simulink library "powerwindowlibdsp"  (Simulink 7.6)
settings: Solver=ode45  SolverMode=SingleTasking  StartTime=0.0  StopTime=10.0  RelTol=1e-3
libraries: powerlib x26, dspquant2 x6, simulink x4, xpclib x2
settings Model: Creator=The MathWorks Inc.  ExtModeAutoUpdateStatusClock=off

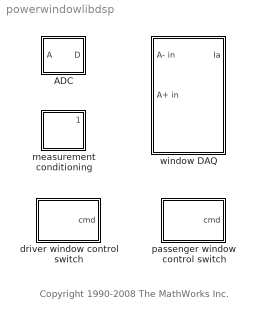
== system powerwindowlibdsp ==
  note: Copyright 1990-2008 The MathWorks Inc.
  ADC : Subsystem  mask(AD Converter){Ts=0.01, peak=3.5, Td=0.005, bits=8}
      mask prompts: Ts "sample time (-1 for inherited)"; Td "delay (-1 for inherited)"
      mask help: Analog (A) to digital (D) converter with sample rate, conversion delay, range, and number of bits used for conversion.
      mask Display:
      | plot([0.5 1.5 1.5 2.5 2.5 3.5 3.5 4.5], [0 0 1 1 2 2 3 3])
      | plot([0 3], [0 3])
  driver window control switch : Subsystem
  measurement conditioning : Subsystem
  passenger window control switch : Subsystem
  window DAQ : Subsystem

== system powerwindowlibdsp/ADC ==
  A : Inport
  Uniform Encoder : dspquant2/Uniform Encoder  peak=peak  bits=bits  otype=Signed integer
  Unit Delay : UnitDelay  SampleTime=Td
  Zero-Order Hold : ZeroOrderHold  SampleTime=Ts
  D : Outport
  wires:
  Uniform Encoder/1 -> D/1
  A/1 -> Unit Delay/1
  Unit Delay/1 -> Zero-Order Hold/1
  Zero-Order Hold/1 -> Uniform Encoder/1

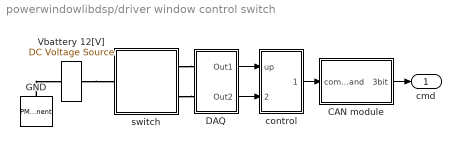
== system powerwindowlibdsp/driver window control switch ==
  CAN module : Subsystem
  DAQ : Subsystem
  GND : PMComponent  PhysicalDomain=powersysdomain  LeftPortType=p1  RightPortType=p1  LConnTagsString=a
      mask Type: Ground
      mask Description: Ground connection.
      mask Help: web(psbhelp);
      mask Display: plot(-10,-10,10,10,-[5 5],[-10 10],[0 0],[-5 5],-[-5 -5],[-2.5 2.5],-[15 5],[0 0])
  Vbattery 12[V] : powerlib/Electrical Sources/DC Voltage Source  SystemSampleTime=-1  Amplitude=12  Measurements=None
  control : Subsystem
  switch : Subsystem
  cmd : Outport
  wires:
  control/1(cmd) -> CAN module/1(command)
  CAN module/1(3bit) -> cmd/1
  DAQ/1(Out1) -> control/1(up)
  DAQ/2(Out2) -> control/2(down)
  connections:
  switch/RConn1 -- DAQ/LConn1
  switch/RConn2 -- DAQ/LConn2
  GND/LConn1 -- Vbattery 12[V]/LConn1
  Vbattery 12[V]/RConn1 -- switch/LConn1

== system powerwindowlibdsp/measurement conditioning ==
  R1 : powerlib/Elements/Series RLC Branch  DialogController=POWERSYS.PowerSysDialog  PhysicalDomain=powersysdomain  SubClassName=unknown  LeftPortType=p1  RightPortType=p1  LConnTagsString=__new0  RConnTagsString=__new0  BranchType=R  Resistance=0.18  Inductance=1.0  SetiL0=off  InitialCurrent=0  Capacitance=1.0  Setx0=off  InitialVoltage=0  Measurements=None
  measure1 : powerlib/Measurements/Voltage Measurement  DialogController=POWERSYS.PowerSysDialog  SystemSampleTime=-1  PhasorSimulation=off  OutputType=Magnitude  PSBequivalent=0
  Vin : PMIOPort  Tag=PMCPort  Port=1  Side=Left
  Vout : PMIOPort  Tag=PMCPort  Port=2  Side=Right
  Vmeas : Outport
  wires:
  measure1/1 -> Vmeas/1
  connections:
  Vout/RConn1 -- measure1/LConn2 -- R1/RConn1
  Vin/RConn1 -- R1/LConn1 -- measure1/LConn1

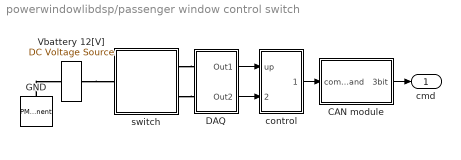
== system powerwindowlibdsp/passenger window control switch ==
  CAN module : Subsystem
  DAQ : Subsystem
  GND : PMComponent  PhysicalDomain=powersysdomain  LeftPortType=p1  RightPortType=p1  LConnTagsString=a
      mask Type: Ground
      mask Description: Ground connection.
      mask Help: web(psbhelp);
      mask Display: plot(-10,-10,10,10,-[5 5],[-10 10],[0 0],[-5 5],-[-5 -5],[-2.5 2.5],-[15 5],[0 0])
  Vbattery 12[V] : powerlib/Electrical Sources/DC Voltage Source  SystemSampleTime=-1  Amplitude=12  Measurements=None
  control : Subsystem
  switch : Subsystem
  cmd : Outport
  wires:
  DAQ/2(Out2) -> control/2(down)
  DAQ/1(Out1) -> control/1(up)
  CAN module/1(3bit) -> cmd/1
  control/1(cmd) -> CAN module/1(command)
  connections:
  Vbattery 12[V]/RConn1 -- switch/LConn1
  GND/LConn1 -- Vbattery 12[V]/LConn1
  switch/RConn2 -- DAQ/LConn2
  switch/RConn1 -- DAQ/LConn1

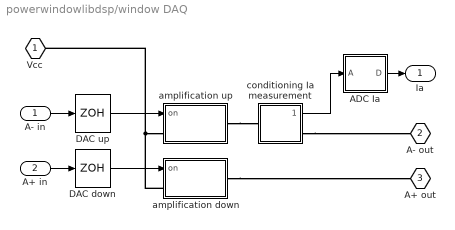
== system powerwindowlibdsp/window DAQ ==
  A- in : Inport
  A+ in : Inport  Port=2
  ADC Ia : Subsystem  mask(AD Converter){Ts=0.01, peak=3.5, Td=0.005, bits=8}
      mask prompts: Ts "sample time (-1 for inherited)"; Td "delay (-1 for inherited)"
      mask help: Analog (A) to digital (D) converter with sample rate, conversion delay, range, and number of bits used for conversion.
      mask Display:
      | plot([0.5 1.5 1.5 2.5 2.5 3.5 3.5 4.5], [0 0 1 1 2 2 3 3])
      | plot([0 3], [0 3])
  DAC down : ZeroOrderHold  SampleTime=0.01
  DAC up : ZeroOrderHold  SampleTime=0.01
  amplification down : Subsystem
  amplification up : Subsystem
  conditioning Ia measurement : Subsystem
  Vcc : PMIOPort  Port=1  Side=Left
  A- out : PMIOPort  Port=2  Side=Right
  A+ out : PMIOPort  Port=3  Side=Right
  Ia : Outport
  wires:
  DAC up/1 -> amplification up/1(on)
  DAC down/1 -> amplification down/1(on)
  conditioning Ia measurement/1(Vmeas) -> ADC Ia/1(A)
  ADC Ia/1(D) -> Ia/1
  A- in/1 -> DAC up/1
  A+ in/1 -> DAC down/1
  connections:
  amplification down/LConn1 -- Vcc/RConn1 -- amplification up/LConn1
  amplification up/RConn1 -- conditioning Ia measurement/LConn1
  conditioning Ia measurement/RConn1 -- A- out/RConn1
  amplification down/RConn1 -- A+ out/RConn1

== system powerwindowlibdsp/driver window control switch/CAN module ==
  command : Inport
  "CAN bit-packing " : xpclib/CAN/Utilities/CAN bit-packing   bitpatterns={ [0:0] [1:1] [2:2]}
  Demux : Demux  Outputs=3
  3bit : Outport
  wires:
  "CAN bit-packing "/1 -> 3bit/1
  command/1 -> Demux/1
  Demux/1 -> "CAN bit-packing "/1
  Demux/2 -> "CAN bit-packing "/2
  Demux/3 -> "CAN bit-packing "/3

== system powerwindowlibdsp/driver window control switch/DAQ ==
  DAQ driver down : Subsystem
  DAQ driver up : Subsystem
  In1 : PMIOPort  Port=1  Side=Left
  In2 : PMIOPort  Port=2  Side=Left
  Out1 : Outport
  Out2 : Outport  Port=2
  wires:
  DAQ driver up/1(active) -> Out1/1
  DAQ driver down/1(active) -> Out2/1
  connections:
  In1/RConn1 -- DAQ driver up/LConn1
  In2/RConn1 -- DAQ driver down/LConn1

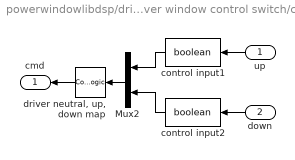
== system powerwindowlibdsp/driver window control switch/control ==
  up : Inport
  down : Inport  Port=2
  Mux2 : Mux  Inputs=2
  control input1 : DataTypeConversion  OutDataTypeStr=boolean  SaturateOnIntegerOverflow=on  RndMeth=Zero
  control input2 : DataTypeConversion  OutDataTypeStr=boolean  SaturateOnIntegerOverflow=on  RndMeth=Zero
  "driver neutral, up, down map" : CombinatorialLogic  TruthTable=[1 0 0;0 0 1;0 1 0;1 0 0]
  cmd : Outport
  wires:
  Mux2/1 -> "driver neutral, up, down map"/1
  control input1/1 -> Mux2/1
  control input2/1 -> Mux2/2
  up/1 -> control input1/1
  "driver neutral, up, down map"/1 -> cmd/1
  down/1 -> control input2/1

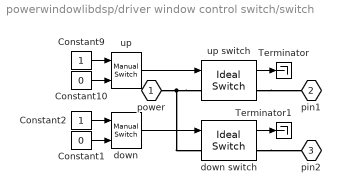
== system powerwindowlibdsp/driver window control switch/switch ==
  Constant1 : Constant  Value=0
  Constant10 : Constant  Value=0
  Constant2 : Constant
  Constant9 : Constant
  Terminator : Terminator
  Terminator1 : Terminator
  down : simulink/Signal Routing/Manual Switch  SystemSampleTime=-1  sw=0  action=0
  down switch : powerlib/Power Electronics/Ideal Switch  SystemSampleTime=-1  Ron=0.01  Lon=0  IC=0  Rs=1000000  Cs=inf  Measurements=on
  up : simulink/Signal Routing/Manual Switch  SystemSampleTime=-1  sw=0  action=0
  up switch : powerlib/Power Electronics/Ideal Switch  SystemSampleTime=-1  Ron=0.01  Lon=0  IC=0  Rs=1000000  Cs=inf  Measurements=on
  power : PMIOPort  Port=1  Side=Left
  pin1 : PMIOPort  Port=2  Side=Right
  pin2 : PMIOPort  Port=3  Side=Right
  wires:
  down/1 -> down switch/1
  down switch/1 -> Terminator1/1
  up/1 -> up switch/1
  up switch/1 -> Terminator/1
  Constant1/1 -> down/2
  Constant2/1 -> down/1
  Constant10/1 -> up/2
  Constant9/1 -> up/1
  connections:
  up switch/LConn1 -- power/RConn1 -- down switch/LConn1
  down switch/RConn1 -- pin2/RConn1
  up switch/RConn1 -- pin1/RConn1

== system powerwindowlibdsp/passenger window control switch/CAN module ==
  command : Inport
  "CAN bit-packing " : xpclib/CAN/Utilities/CAN bit-packing   bitpatterns={ [0:0] [1:1] [2:2]}
  Demux : Demux  Outputs=3
  3bit : Outport
  wires:
  Demux/3 -> "CAN bit-packing "/3
  Demux/2 -> "CAN bit-packing "/2
  Demux/1 -> "CAN bit-packing "/1
  command/1 -> Demux/1
  "CAN bit-packing "/1 -> 3bit/1

== system powerwindowlibdsp/passenger window control switch/DAQ ==
  DAQ driver down : Subsystem
  DAQ driver up : Subsystem
  In1 : PMIOPort  Port=1  Side=Left
  In2 : PMIOPort  Port=2  Side=Left
  Out1 : Outport
  Out2 : Outport  Port=2
  wires:
  DAQ driver down/1(active) -> Out2/1
  DAQ driver up/1(active) -> Out1/1
  connections:
  In2/RConn1 -- DAQ driver down/LConn1
  In1/RConn1 -- DAQ driver up/LConn1

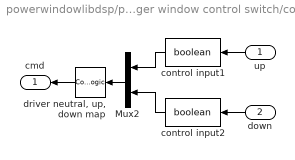
== system powerwindowlibdsp/passenger window control switch/control ==
  up : Inport
  down : Inport  Port=2
  Mux2 : Mux  Inputs=2
  control input1 : DataTypeConversion  OutDataTypeStr=boolean  SaturateOnIntegerOverflow=on  RndMeth=Zero
  control input2 : DataTypeConversion  OutDataTypeStr=boolean  SaturateOnIntegerOverflow=on  RndMeth=Zero
  "driver neutral, up, down map" : CombinatorialLogic  TruthTable=[1 0 0;0 0 1;0 1 0;1 0 0]
  cmd : Outport
  wires:
  down/1 -> control input2/1
  "driver neutral, up, down map"/1 -> cmd/1
  up/1 -> control input1/1
  control input2/1 -> Mux2/2
  control input1/1 -> Mux2/1
  Mux2/1 -> "driver neutral, up, down map"/1

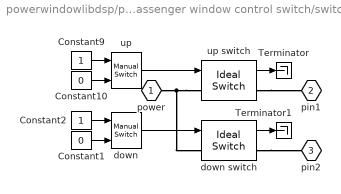
== system powerwindowlibdsp/passenger window control switch/switch ==
  Constant1 : Constant  Value=0
  Constant10 : Constant  Value=0
  Constant2 : Constant
  Constant9 : Constant
  Terminator : Terminator
  Terminator1 : Terminator
  down : simulink/Signal Routing/Manual Switch  SystemSampleTime=-1  sw=0  action=0
  down switch : powerlib/Power Electronics/Ideal Switch  SystemSampleTime=-1  Ron=0.01  Lon=0  IC=0  Rs=1000000  Cs=inf  Measurements=on
  up : simulink/Signal Routing/Manual Switch  SystemSampleTime=-1  sw=0  action=0
  up switch : powerlib/Power Electronics/Ideal Switch  SystemSampleTime=-1  Ron=0.01  Lon=0  IC=0  Rs=1000000  Cs=inf  Measurements=on
  power : PMIOPort  Port=1  Side=Left
  pin1 : PMIOPort  Port=2  Side=Right
  pin2 : PMIOPort  Port=3  Side=Right
  wires:
  Constant9/1 -> up/1
  Constant10/1 -> up/2
  Constant2/1 -> down/1
  Constant1/1 -> down/2
  up switch/1 -> Terminator/1
  up/1 -> up switch/1
  down switch/1 -> Terminator1/1
  down/1 -> down switch/1
  connections:
  up switch/RConn1 -- pin1/RConn1
  down switch/RConn1 -- pin2/RConn1
  up switch/LConn1 -- down switch/LConn1 -- power/RConn1

== system powerwindowlibdsp/window DAQ/ADC Ia ==
  A : Inport
  Uniform Encoder : dspquant2/Uniform Encoder  peak=peak  bits=bits  otype=Signed integer
  Unit Delay : UnitDelay  SampleTime=Td
  Zero-Order Hold : ZeroOrderHold  SampleTime=Ts
  D : Outport
  wires:
  Uniform Encoder/1 -> D/1
  A/1 -> Unit Delay/1
  Unit Delay/1 -> Zero-Order Hold/1
  Zero-Order Hold/1 -> Uniform Encoder/1

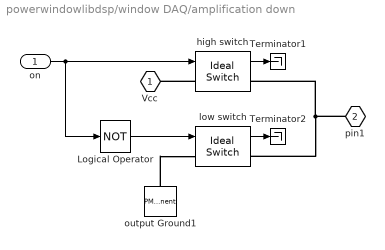
== system powerwindowlibdsp/window DAQ/amplification down ==
  on : Inport
  Logical Operator : Logic  Operator=NOT
  Terminator1 : Terminator
  Terminator2 : Terminator
  high switch : powerlib/Power Electronics/Ideal Switch  DialogController=POWERSYS.PowerSysDialog  SystemSampleTime=-1  Ron=0.01  Lon=0  IC=0  Rs=1000000  Cs=inf  Measurements=on
  low switch : powerlib/Power Electronics/Ideal Switch  DialogController=POWERSYS.PowerSysDialog  SystemSampleTime=-1  Ron=0.01  Lon=0  IC=0  Rs=1000000  Cs=inf  Measurements=on
  output Ground1 : PMComponent  PhysicalDomain=powersysdomain  LeftPortType=p1  RightPortType=p1  LConnTagsString=a
      mask Type: Ground
      mask Description: Ground connection.
      mask Help: web(psbhelp);
      mask Display: plot(-10,-10,10,10,-[5 5],[-10 10],[0 0],[-5 5],-[-5 -5],[-2.5 2.5],-[15 5],[0 0])
  Vcc : PMIOPort  Port=1  Side=Left
  pin1 : PMIOPort  Port=2  Side=Right
  wires:
  low switch/1 -> Terminator2/1
  on/1 -> Logical Operator/1, high switch/1
  high switch/1 -> Terminator1/1
  Logical Operator/1 -> low switch/1
  connections:
  high switch/LConn1 -- Vcc/RConn1
  output Ground1/LConn1 -- low switch/LConn1
  low switch/RConn1 -- high switch/RConn1 -- pin1/RConn1

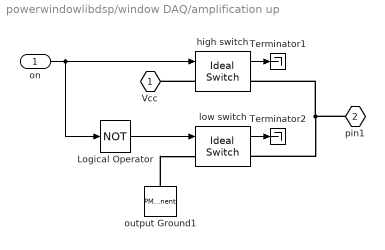
== system powerwindowlibdsp/window DAQ/amplification up ==
  on : Inport
  Logical Operator : Logic  Operator=NOT
  Terminator1 : Terminator
  Terminator2 : Terminator
  high switch : powerlib/Power Electronics/Ideal Switch  DialogController=POWERSYS.PowerSysDialog  SystemSampleTime=-1  Ron=0.01  Lon=0  IC=0  Rs=1000000  Cs=inf  Measurements=on
  low switch : powerlib/Power Electronics/Ideal Switch  SystemSampleTime=-1  Ron=0.01  Lon=0  IC=0  Rs=1000000  Cs=inf  Measurements=on
  output Ground1 : PMComponent  PhysicalDomain=powersysdomain  LeftPortType=p1  RightPortType=p1  LConnTagsString=a
      mask Type: Ground
      mask Description: Ground connection.
      mask Help: web(psbhelp);
      mask Display: plot(-10,-10,10,10,-[5 5],[-10 10],[0 0],[-5 5],-[-5 -5],[-2.5 2.5],-[15 5],[0 0])
  Vcc : PMIOPort  Port=1  Side=Left
  pin1 : PMIOPort  Port=2  Side=Right
  wires:
  low switch/1 -> Terminator2/1
  on/1 -> high switch/1, Logical Operator/1
  high switch/1 -> Terminator1/1
  Logical Operator/1 -> low switch/1
  connections:
  high switch/RConn1 -- low switch/RConn1 -- pin1/RConn1
  high switch/LConn1 -- Vcc/RConn1
  output Ground1/LConn1 -- low switch/LConn1

== system powerwindowlibdsp/window DAQ/conditioning Ia measurement ==
  R1 : powerlib/Elements/Series RLC Branch  DialogController=POWERSYS.PowerSysDialog  PhysicalDomain=powersysdomain  SubClassName=unknown  LeftPortType=p1  RightPortType=p1  LConnTagsString=__new0  RConnTagsString=__new0  BranchType=R  Resistance=0.18  Inductance=1.0  SetiL0=off  InitialCurrent=0  Capacitance=1.0  Setx0=off  InitialVoltage=0  Measurements=None
  measure1 : powerlib/Measurements/Voltage Measurement  DialogController=POWERSYS.PowerSysDialog  SystemSampleTime=-1  PhasorSimulation=off  OutputType=Magnitude  PSBequivalent=0
  Vin : PMIOPort  Port=1  Side=Left
  Vout : PMIOPort  Port=2  Side=Right
  Vmeas : Outport
  wires:
  measure1/1 -> Vmeas/1
  connections:
  measure1/LConn2 -- Vout/RConn1 -- R1/RConn1
  R1/LConn1 -- measure1/LConn1 -- Vin/RConn1

== system powerwindowlibdsp/driver window control switch/DAQ/DAQ driver down ==
  ADC driver up : Subsystem  mask(AD Converter){Ts=0.01, Td=0.005, peak=4.9, bits=2}
      mask prompts: Ts "sample time (-1 for inherited)"; Td "delay (-1 for inherited)"
      mask help: Analog (A) to digital (D) converter with sample rate, conversion delay, range, and number of bits used for conversion.
      mask init:
      | gain = peak / (2^(bits-1));
      mask Display:
      | plot([0.5 1.5 1.5 2.5 2.5 3.5 3.5 4.5], [0 0 1 1 2 2 3 3])
      | plot([0 3], [0 3])
  conditioning driver up : Subsystem
  Vin : PMIOPort  Port=1  Side=Left
  active : Outport
  wires:
  ADC driver up/1(D) -> active/1
  conditioning driver up/1(active) -> ADC driver up/1(A)
  connections:
  Vin/RConn1 -- conditioning driver up/LConn1

== system powerwindowlibdsp/driver window control switch/DAQ/DAQ driver up ==
  ADC driver up : Subsystem  mask(AD Converter){Ts=0.01, Td=0.005, peak=4.9, bits=2}
      mask prompts: Ts "sample time (-1 for inherited)"; Td "delay (-1 for inherited)"
      mask help: Analog (A) to digital (D) converter with sample rate, conversion delay, range, and number of bits used for conversion.
      mask init:
      | gain = peak / (2^(bits-1));
      mask Display:
      | plot([0.5 1.5 1.5 2.5 2.5 3.5 3.5 4.5], [0 0 1 1 2 2 3 3])
      | plot([0 3], [0 3])
  conditioning driver up : Subsystem
  Vin : PMIOPort  Port=1  Side=Left
  active : Outport
  wires:
  conditioning driver up/1(active) -> ADC driver up/1(A)
  ADC driver up/1(D) -> active/1
  connections:
  Vin/RConn1 -- conditioning driver up/LConn1

== system powerwindowlibdsp/passenger window control switch/DAQ/DAQ driver down ==
  ADC driver up : Subsystem  mask(AD Converter){Ts=0.01, Td=0.005, peak=4.9, bits=2}
      mask prompts: Ts "sample time (-1 for inherited)"; Td "delay (-1 for inherited)"
      mask help: Analog (A) to digital (D) converter with sample rate, conversion delay, range, and number of bits used for conversion.
      mask init:
      | gain = peak / (2^(bits-1));
      mask Display:
      | plot([0.5 1.5 1.5 2.5 2.5 3.5 3.5 4.5], [0 0 1 1 2 2 3 3])
      | plot([0 3], [0 3])
  conditioning driver up : Subsystem
  Vin : PMIOPort  Port=1  Side=Left
  active : Outport
  wires:
  conditioning driver up/1(active) -> ADC driver up/1(A)
  ADC driver up/1(D) -> active/1
  connections:
  Vin/RConn1 -- conditioning driver up/LConn1

== system powerwindowlibdsp/passenger window control switch/DAQ/DAQ driver up ==
  ADC driver up : Subsystem  mask(AD Converter){Ts=0.01, Td=0.005, peak=4.9, bits=2}
      mask prompts: Ts "sample time (-1 for inherited)"; Td "delay (-1 for inherited)"
      mask help: Analog (A) to digital (D) converter with sample rate, conversion delay, range, and number of bits used for conversion.
      mask init:
      | gain = peak / (2^(bits-1));
      mask Display:
      | plot([0.5 1.5 1.5 2.5 2.5 3.5 3.5 4.5], [0 0 1 1 2 2 3 3])
      | plot([0 3], [0 3])
  conditioning driver up : Subsystem
  Vin : PMIOPort  Port=1  Side=Left
  active : Outport
  wires:
  ADC driver up/1(D) -> active/1
  conditioning driver up/1(active) -> ADC driver up/1(A)
  connections:
  Vin/RConn1 -- conditioning driver up/LConn1

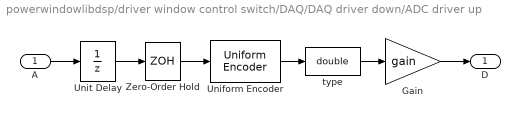
== system powerwindowlibdsp/driver window control switch/DAQ/DAQ driver down/ADC driver up ==
  A : Inport
  Gain : Gain  Gain=gain  SaturateOnIntegerOverflow=on  OutDataTypeStr=Inherit: Same as input  ParamDataTypeStr=Inherit: Same as input
  Uniform Encoder : dspquant2/Uniform Encoder  peak=peak  bits=bits  otype=Signed integer
  Unit Delay : UnitDelay  SampleTime=Td
  Zero-Order Hold : ZeroOrderHold  SampleTime=Ts
  type : DataTypeConversion  OutDataTypeStr=double  SaturateOnIntegerOverflow=on  RndMeth=Zero
  D : Outport
  wires:
  Zero-Order Hold/1 -> Uniform Encoder/1
  Unit Delay/1 -> Zero-Order Hold/1
  A/1 -> Unit Delay/1
  Uniform Encoder/1 -> type/1
  type/1 -> Gain/1
  Gain/1 -> D/1

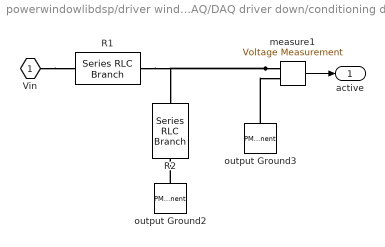
== system powerwindowlibdsp/driver window control switch/DAQ/DAQ driver down/conditioning driver up ==
  R1 : powerlib/Elements/Series RLC Branch  PhysicalDomain=powersysdomain  SubClassName=unknown  LeftPortType=p1  RightPortType=p1  LConnTagsString=__new0  RConnTagsString=__new0  BranchType=R  Resistance=6800  Inductance=1.0  SetiL0=off  InitialCurrent=0  Capacitance=1.0  Setx0=off  InitialVoltage=0  Measurements=None
  R2 : powerlib/Elements/Series RLC Branch  PhysicalDomain=powersysdomain  SubClassName=unknown  LeftPortType=p1  RightPortType=p1  LConnTagsString=__new0  RConnTagsString=__new0  BranchType=R  Resistance=4700  Inductance=1.0  SetiL0=off  InitialCurrent=0  Capacitance=1.0  Setx0=off  InitialVoltage=0  Measurements=None
  measure1 : powerlib/Measurements/Voltage Measurement  SystemSampleTime=-1  PhasorSimulation=off  OutputType=Magnitude  PSBequivalent=0
  output Ground2 : PMComponent  PhysicalDomain=powersysdomain  LeftPortType=p1  RightPortType=p1  LConnTagsString=a
      mask Type: Ground
      mask Description: Ground connection.
      mask Help: web(psbhelp);
      mask Display: plot(-10,-10,10,10,-[5 5],[-10 10],[0 0],[-5 5],-[-5 -5],[-2.5 2.5],-[15 5],[0 0])
  output Ground3 : PMComponent  PhysicalDomain=powersysdomain  LeftPortType=p1  RightPortType=p1  LConnTagsString=a
      mask Type: Ground
      mask Description: Ground connection.
      mask Help: web(psbhelp);
      mask Display: plot(-10,-10,10,10,-[5 5],[-10 10],[0 0],[-5 5],-[-5 -5],[-2.5 2.5],-[15 5],[0 0])
  Vin : PMIOPort  Port=1  Side=Left
  active : Outport
  wires:
  measure1/1 -> active/1
  connections:
  output Ground3/LConn1 -- measure1/LConn2
  output Ground2/LConn1 -- R2/LConn1
  Vin/RConn1 -- R1/LConn1
  measure1/LConn1 -- R2/RConn1 -- R1/RConn1

== system powerwindowlibdsp/driver window control switch/DAQ/DAQ driver up/ADC driver up ==
  A : Inport
  Gain : Gain  Gain=gain  SaturateOnIntegerOverflow=on  OutDataTypeStr=Inherit: Same as input  ParamDataTypeStr=Inherit: Same as input
  Uniform Encoder : dspquant2/Uniform Encoder  peak=peak  bits=bits  otype=Signed integer
  Unit Delay : UnitDelay  SampleTime=Td
  Zero-Order Hold : ZeroOrderHold  SampleTime=Ts
  type : DataTypeConversion  OutDataTypeStr=double  SaturateOnIntegerOverflow=on  RndMeth=Zero
  D : Outport
  wires:
  Gain/1 -> D/1
  type/1 -> Gain/1
  Uniform Encoder/1 -> type/1
  A/1 -> Unit Delay/1
  Unit Delay/1 -> Zero-Order Hold/1
  Zero-Order Hold/1 -> Uniform Encoder/1

== system powerwindowlibdsp/driver window control switch/DAQ/DAQ driver up/conditioning driver up ==
  R1 : powerlib/Elements/Series RLC Branch  PhysicalDomain=powersysdomain  SubClassName=unknown  LeftPortType=p1  RightPortType=p1  LConnTagsString=__new0  RConnTagsString=__new0  BranchType=R  Resistance=6800  Inductance=1.0  SetiL0=off  InitialCurrent=0  Capacitance=1.0  Setx0=off  InitialVoltage=0  Measurements=None
  R2 : powerlib/Elements/Series RLC Branch  PhysicalDomain=powersysdomain  SubClassName=unknown  LeftPortType=p1  RightPortType=p1  LConnTagsString=__new0  RConnTagsString=__new0  BranchType=R  Resistance=4700  Inductance=1.0  SetiL0=off  InitialCurrent=0  Capacitance=1.0  Setx0=off  InitialVoltage=0  Measurements=None
  measure1 : powerlib/Measurements/Voltage Measurement  SystemSampleTime=-1  PhasorSimulation=off  OutputType=Magnitude  PSBequivalent=0
  output Ground2 : PMComponent  PhysicalDomain=powersysdomain  LeftPortType=p1  RightPortType=p1  LConnTagsString=a
      mask Type: Ground
      mask Description: Ground connection.
      mask Help: web(psbhelp);
      mask Display: plot(-10,-10,10,10,-[5 5],[-10 10],[0 0],[-5 5],-[-5 -5],[-2.5 2.5],-[15 5],[0 0])
  output Ground3 : PMComponent  PhysicalDomain=powersysdomain  LeftPortType=p1  RightPortType=p1  LConnTagsString=a
      mask Type: Ground
      mask Description: Ground connection.
      mask Help: web(psbhelp);
      mask Display: plot(-10,-10,10,10,-[5 5],[-10 10],[0 0],[-5 5],-[-5 -5],[-2.5 2.5],-[15 5],[0 0])
  Vin : PMIOPort  Port=1  Side=Left
  active : Outport
  wires:
  measure1/1 -> active/1
  connections:
  measure1/LConn1 -- R1/RConn1 -- R2/RConn1
  Vin/RConn1 -- R1/LConn1
  output Ground2/LConn1 -- R2/LConn1
  output Ground3/LConn1 -- measure1/LConn2

== system powerwindowlibdsp/passenger window control switch/DAQ/DAQ driver down/ADC driver up ==
  A : Inport
  Gain : Gain  Gain=gain  SaturateOnIntegerOverflow=on  OutDataTypeStr=Inherit: Same as input  ParamDataTypeStr=Inherit: Same as input
  Uniform Encoder : dspquant2/Uniform Encoder  peak=peak  bits=bits  otype=Signed integer
  Unit Delay : UnitDelay  SampleTime=Td
  Zero-Order Hold : ZeroOrderHold  SampleTime=Ts
  type : DataTypeConversion  OutDataTypeStr=double  SaturateOnIntegerOverflow=on  RndMeth=Zero
  D : Outport
  wires:
  Gain/1 -> D/1
  type/1 -> Gain/1
  Uniform Encoder/1 -> type/1
  A/1 -> Unit Delay/1
  Unit Delay/1 -> Zero-Order Hold/1
  Zero-Order Hold/1 -> Uniform Encoder/1

== system powerwindowlibdsp/passenger window control switch/DAQ/DAQ driver down/conditioning driver up ==
  R1 : powerlib/Elements/Series RLC Branch  PhysicalDomain=powersysdomain  SubClassName=unknown  LeftPortType=p1  RightPortType=p1  LConnTagsString=__new0  RConnTagsString=__new0  BranchType=R  Resistance=6800  Inductance=1.0  SetiL0=off  InitialCurrent=0  Capacitance=1.0  Setx0=off  InitialVoltage=0  Measurements=None
  R2 : powerlib/Elements/Series RLC Branch  PhysicalDomain=powersysdomain  SubClassName=unknown  LeftPortType=p1  RightPortType=p1  LConnTagsString=__new0  RConnTagsString=__new0  BranchType=R  Resistance=4700  Inductance=1.0  SetiL0=off  InitialCurrent=0  Capacitance=1.0  Setx0=off  InitialVoltage=0  Measurements=None
  measure1 : powerlib/Measurements/Voltage Measurement  SystemSampleTime=-1  PhasorSimulation=off  OutputType=Magnitude  PSBequivalent=0
  output Ground2 : PMComponent  PhysicalDomain=powersysdomain  LeftPortType=p1  RightPortType=p1  LConnTagsString=a
      mask Type: Ground
      mask Description: Ground connection.
      mask Help: web(psbhelp);
      mask Display: plot(-10,-10,10,10,-[5 5],[-10 10],[0 0],[-5 5],-[-5 -5],[-2.5 2.5],-[15 5],[0 0])
  output Ground3 : PMComponent  PhysicalDomain=powersysdomain  LeftPortType=p1  RightPortType=p1  LConnTagsString=a
      mask Type: Ground
      mask Description: Ground connection.
      mask Help: web(psbhelp);
      mask Display: plot(-10,-10,10,10,-[5 5],[-10 10],[0 0],[-5 5],-[-5 -5],[-2.5 2.5],-[15 5],[0 0])
  Vin : PMIOPort  Port=1  Side=Left
  active : Outport
  wires:
  measure1/1 -> active/1
  connections:
  R1/RConn1 -- R2/RConn1 -- measure1/LConn1
  Vin/RConn1 -- R1/LConn1
  output Ground2/LConn1 -- R2/LConn1
  output Ground3/LConn1 -- measure1/LConn2

== system powerwindowlibdsp/passenger window control switch/DAQ/DAQ driver up/ADC driver up ==
  A : Inport
  Gain : Gain  Gain=gain  SaturateOnIntegerOverflow=on  OutDataTypeStr=Inherit: Same as input  ParamDataTypeStr=Inherit: Same as input
  Uniform Encoder : dspquant2/Uniform Encoder  peak=peak  bits=bits  otype=Signed integer
  Unit Delay : UnitDelay  SampleTime=Td
  Zero-Order Hold : ZeroOrderHold  SampleTime=Ts
  type : DataTypeConversion  OutDataTypeStr=double  SaturateOnIntegerOverflow=on  RndMeth=Zero
  D : Outport
  wires:
  Zero-Order Hold/1 -> Uniform Encoder/1
  Unit Delay/1 -> Zero-Order Hold/1
  A/1 -> Unit Delay/1
  Uniform Encoder/1 -> type/1
  type/1 -> Gain/1
  Gain/1 -> D/1

== system powerwindowlibdsp/passenger window control switch/DAQ/DAQ driver up/conditioning driver up ==
  R1 : powerlib/Elements/Series RLC Branch  PhysicalDomain=powersysdomain  SubClassName=unknown  LeftPortType=p1  RightPortType=p1  LConnTagsString=__new0  RConnTagsString=__new0  BranchType=R  Resistance=6800  Inductance=1.0  SetiL0=off  InitialCurrent=0  Capacitance=1.0  Setx0=off  InitialVoltage=0  Measurements=None
  R2 : powerlib/Elements/Series RLC Branch  PhysicalDomain=powersysdomain  SubClassName=unknown  LeftPortType=p1  RightPortType=p1  LConnTagsString=__new0  RConnTagsString=__new0  BranchType=R  Resistance=4700  Inductance=1.0  SetiL0=off  InitialCurrent=0  Capacitance=1.0  Setx0=off  InitialVoltage=0  Measurements=None
  measure1 : powerlib/Measurements/Voltage Measurement  SystemSampleTime=-1  PhasorSimulation=off  OutputType=Magnitude  PSBequivalent=0
  output Ground2 : PMComponent  PhysicalDomain=powersysdomain  LeftPortType=p1  RightPortType=p1  LConnTagsString=a
      mask Type: Ground
      mask Description: Ground connection.
      mask Help: web(psbhelp);
      mask Display: plot(-10,-10,10,10,-[5 5],[-10 10],[0 0],[-5 5],-[-5 -5],[-2.5 2.5],-[15 5],[0 0])
  output Ground3 : PMComponent  PhysicalDomain=powersysdomain  LeftPortType=p1  RightPortType=p1  LConnTagsString=a
      mask Type: Ground
      mask Description: Ground connection.
      mask Help: web(psbhelp);
      mask Display: plot(-10,-10,10,10,-[5 5],[-10 10],[0 0],[-5 5],-[-5 -5],[-2.5 2.5],-[15 5],[0 0])
  Vin : PMIOPort  Port=1  Side=Left
  active : Outport
  wires:
  measure1/1 -> active/1
  connections:
  output Ground3/LConn1 -- measure1/LConn2
  output Ground2/LConn1 -- R2/LConn1
  Vin/RConn1 -- R1/LConn1
  measure1/LConn1 -- R2/RConn1 -- R1/RConn1
